simulink model "dynamic_calc"  (R2022b)
settings: Solver=VariableStepAuto  StartTime=0.0  StopTime=10.0  RelTol=1e-3
undefined symbols (not defined in the file): alfa_1, gravity_acceleration, i, Malpha, Malphadot, MdeltaE, Mq, Mtalpha, Mtu, Mu, o, Vp1, Xalpha, XdeltaE, Xtu, Xu, Zalpha, Zalphadot, ZdeltaE, Zq, Zu
libraries: simulink_extras x3
settings Model: Creator=48519  LastModifiedBy=48519

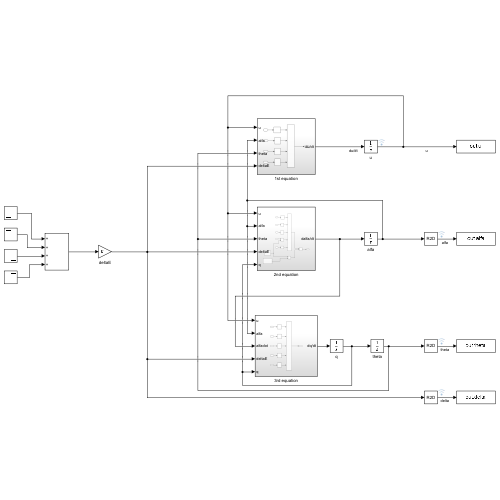
[thumbnail: Simulink's stored preview of the top-level diagram]
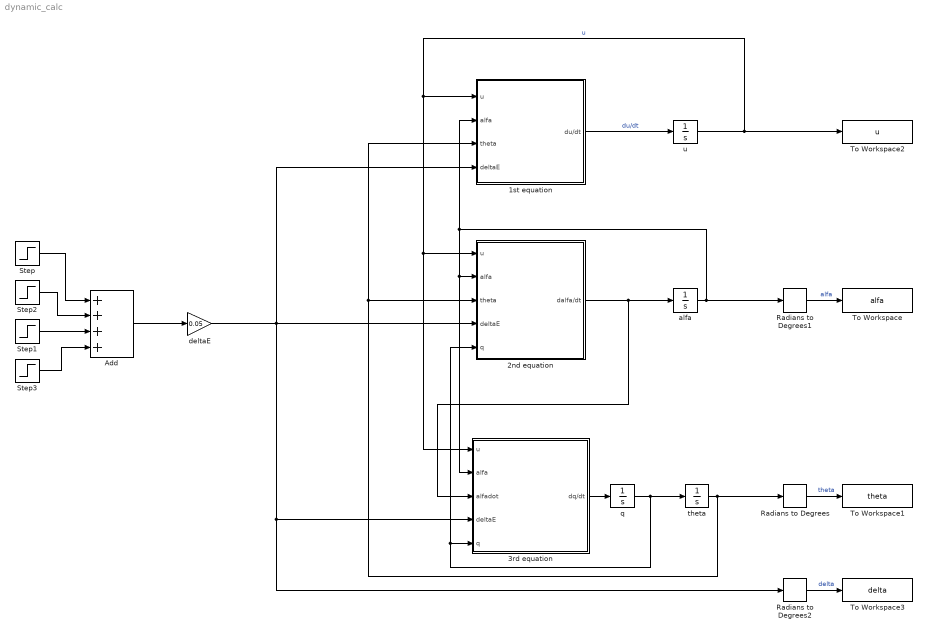
== system dynamic_calc ==
  1st equation : Subsystem
  2nd equation : Subsystem
  3rd equation : Subsystem
  Add : Sum  Inputs=++++
  Radians to Degrees : simulink_extras/Transformations/Radians to Degrees
  Radians to Degrees1 : simulink_extras/Transformations/Radians to Degrees
  Radians to Degrees2 : simulink_extras/Transformations/Radians to Degrees
  Step : Step  Time=2  SampleTime=0
  Step1 : Step  Time=62  After=-1  SampleTime=0
  Step2 : Step  Time=7  After=-1  SampleTime=0
  Step3 : Step  Time=67  SampleTime=0
  To Workspace : ToWorkspace  VariableName=alfa  SaveFormat=Timeseries  SampleTime=-1
  To Workspace1 : ToWorkspace  VariableName=theta  SaveFormat=Timeseries  SampleTime=-1
  To Workspace2 : ToWorkspace  VariableName=u  SaveFormat=Timeseries  SampleTime=-1
  To Workspace3 : ToWorkspace  VariableName=delta  SaveFormat=Timeseries  SampleTime=-1
  alfa : Integrator
  deltaE : Gain  Gain=0.05
  q : Integrator
  theta : Integrator
  u : Integrator
  wires:
  Radians to Degrees/1 -> To Workspace1/1  "theta"
  Radians to Degrees2/1 -> To Workspace3/1  "delta"
  theta/1 -> Radians to Degrees/1, 1st equation/3(theta), 2nd equation/3(theta)
  1st equation/1(du/dt) -> u/1  "du/dt"
  alfa/1 -> 3rd equation/2(alfa), 2nd equation/2(alfa), 1st equation/2(alfa), Radians to Degrees1/1
  Step1/1 -> Add/3
  deltaE/1 -> Radians to Degrees2/1, 3rd equation/4(deltaE), 1st equation/4(deltaE), 2nd equation/4(deltaE)
  3rd equation/1(dq/dt) -> q/1
  Step2/1 -> Add/2
  Step/1 -> Add/1
  u/1 -> 2nd equation/1(u), 3rd equation/1(u), 1st equation/1(u), To Workspace2/1  "u"
  Radians to Degrees1/1 -> To Workspace/1  "alfa"
  Step3/1 -> Add/4
  Add/1 -> deltaE/1
  q/1 -> theta/1, 3rd equation/5(q), 2nd equation/5(q)
  2nd equation/1(dalfa/dt) -> 3rd equation/3(alfadot), alfa/1

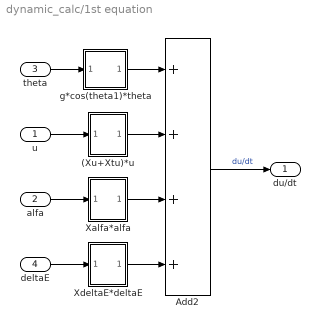
== system dynamic_calc/1st equation ==
  u : Inport
  alfa : Inport  Port=2
  theta : Inport  Port=3
  deltaE : Inport  Port=4
  (Xu+Xtu)*u : Subsystem
  Add2 : Sum  Inputs=++++
  Xalfa*alfa : Subsystem
  XdeltaE*deltaE : Subsystem
  g*cos(theta1)*theta : Subsystem
  du/dt : Outport
  wires:
  Add2/1 -> du/dt/1  "du/dt"
  theta/1 -> g*cos(theta1)*theta/1(theta)
  g*cos(theta1)*theta/1(Out1) -> Add2/1
  u/1 -> (Xu+Xtu)*u/1(In2)
  (Xu+Xtu)*u/1(Out1) -> Add2/2
  alfa/1 -> Xalfa*alfa/1(In1)
  Xalfa*alfa/1(Out1) -> Add2/3
  deltaE/1 -> XdeltaE*deltaE/1(In1)
  XdeltaE*deltaE/1(Out1) -> Add2/4

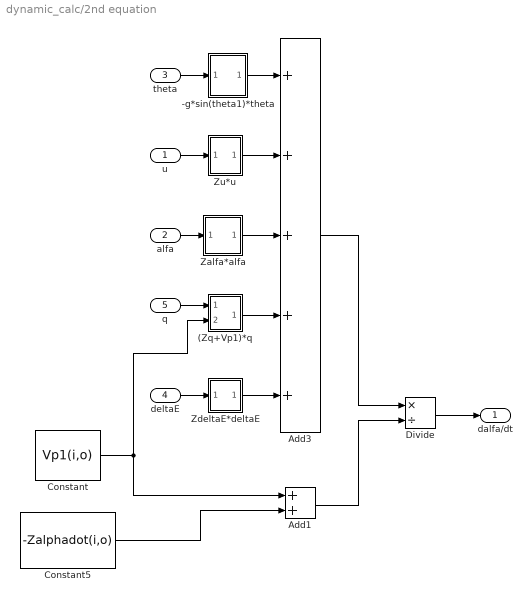
== system dynamic_calc/2nd equation ==
  u : Inport
  alfa : Inport  Port=2
  theta : Inport  Port=3
  deltaE : Inport  Port=4
  q : Inport  Port=5
  (Zq+Vp1)*q : Subsystem
  -g*sin(theta1)*theta : Subsystem
  Add1 : Sum
  Add3 : Sum  Inputs=+++++
  Constant : Constant  Value=Vp1(i,o)
  Constant5 : Constant  Value=-Zalphadot(i,o)
  Divide : Product  Inputs=*/
  Zalfa*alfa : Subsystem
  ZdeltaE*deltaE : Subsystem
  Zu*u : Subsystem
  dalfa/dt : Outport
  wires:
  Constant5/1 -> Add1/2
  Constant/1 -> Add1/1, (Zq+Vp1)*q/2(In2)
  Add3/1 -> Divide/1
  Add1/1 -> Divide/2
  Divide/1 -> dalfa/dt/1
  theta/1 -> -g*sin(theta1)*theta/1(In3)
  -g*sin(theta1)*theta/1(Out1) -> Add3/1
  u/1 -> Zu*u/1(In2)
  Zu*u/1(Out1) -> Add3/2
  alfa/1 -> Zalfa*alfa/1(In1)
  Zalfa*alfa/1(Out1) -> Add3/3
  q/1 -> (Zq+Vp1)*q/1(In5)
  (Zq+Vp1)*q/1(Out1) -> Add3/4
  deltaE/1 -> ZdeltaE*deltaE/1(In4)
  ZdeltaE*deltaE/1(Out1) -> Add3/5

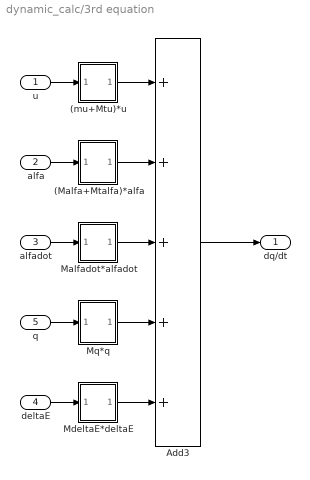
== system dynamic_calc/3rd equation ==
  u : Inport
  alfa : Inport  Port=2
  alfadot : Inport  Port=3
  deltaE : Inport  Port=4
  q : Inport  Port=5
  (Malfa+Mtalfa)*alfa : Subsystem
  (mu+Mtu)*u : Subsystem
  Add3 : Sum  Inputs=+++++
  Malfadot*alfadot : Subsystem
  MdeltaE*deltaE : Subsystem
  Mq*q : Subsystem
  dq/dt : Outport
  wires:
  Add3/1 -> dq/dt/1
  u/1 -> (mu+Mtu)*u/1(In1)
  (mu+Mtu)*u/1(Out1) -> Add3/1
  alfa/1 -> (Malfa+Mtalfa)*alfa/1(In3)
  (Malfa+Mtalfa)*alfa/1(Out1) -> Add3/2
  alfadot/1 -> Malfadot*alfadot/1(In2)
  Malfadot*alfadot/1(Out1) -> Add3/3
  q/1 -> Mq*q/1(In5)
  Mq*q/1(Out1) -> Add3/4
  deltaE/1 -> MdeltaE*deltaE/1(In4)
  MdeltaE*deltaE/1(Out1) -> Add3/5

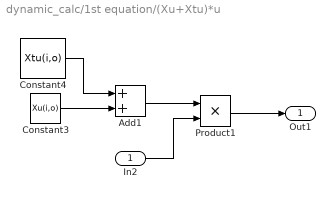
== system dynamic_calc/1st equation/(Xu+Xtu)*u ==
  In2 : Inport
  Add1 : Sum
  Constant3 : Constant  Value=Xu(i,o)
  Constant4 : Constant  Value=Xtu(i,o)
  Product1 : Product
  Out1 : Outport
  wires:
  Constant3/1 -> Add1/2
  Product1/1 -> Out1/1
  Constant4/1 -> Add1/1
  In2/1 -> Product1/2
  Add1/1 -> Product1/1

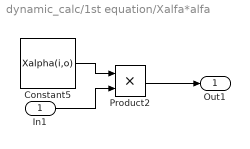
== system dynamic_calc/1st equation/Xalfa*alfa ==
  In1 : Inport
  Constant5 : Constant  Value=Xalpha(i,o)
  Product2 : Product
  Out1 : Outport
  wires:
  Constant5/1 -> Product2/1
  Product2/1 -> Out1/1
  In1/1 -> Product2/2

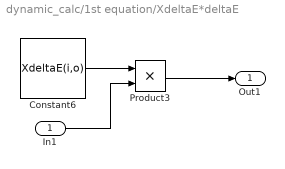
== system dynamic_calc/1st equation/XdeltaE*deltaE ==
  In1 : Inport
  Constant6 : Constant  Value=XdeltaE(i,o)
  Product3 : Product
  Out1 : Outport
  wires:
  Constant6/1 -> Product3/1
  Product3/1 -> Out1/1
  In1/1 -> Product3/2

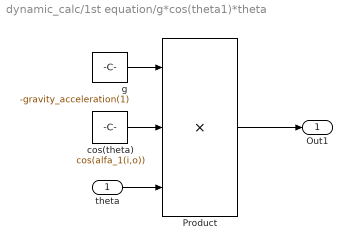
== system dynamic_calc/1st equation/g*cos(theta1)*theta ==
  theta : Inport
  Product : Product  Inputs=3
  cos(theta) : Constant  Value=cos(alfa_1(i,o))
  g : Constant  Value=-gravity_acceleration(1)
  Out1 : Outport
  wires:
  Product/1 -> Out1/1
  g/1 -> Product/1
  theta/1 -> Product/3
  cos(theta)/1 -> Product/2

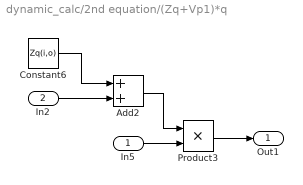
== system dynamic_calc/2nd equation/(Zq+Vp1)*q ==
  In5 : Inport
  In2 : Inport  Port=2
  Add2 : Sum
  Constant6 : Constant  Value=Zq(i,o)
  Product3 : Product
  Out1 : Outport
  wires:
  In2/1 -> Add2/2
  Add2/1 -> Product3/1
  Constant6/1 -> Add2/1
  In5/1 -> Product3/2
  Product3/1 -> Out1/1

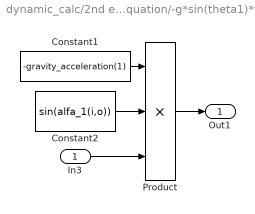
== system dynamic_calc/2nd equation/-g*sin(theta1)*theta ==
  In3 : Inport
  Constant1 : Constant  Value=-gravity_acceleration(1)
  Constant2 : Constant  Value=sin(alfa_1(i,o))
  Product : Product  Inputs=3
  Out1 : Outport
  wires:
  Constant2/1 -> Product/2
  Constant1/1 -> Product/1
  In3/1 -> Product/3
  Product/1 -> Out1/1

== system dynamic_calc/2nd equation/Zalfa*alfa ==
  In1 : Inport
  Constant4 : Constant  Value=Zalpha(i,o)
  Product2 : Product
  Out1 : Outport
  wires:
  Constant4/1 -> Product2/1
  In1/1 -> Product2/2
  Product2/1 -> Out1/1

== system dynamic_calc/2nd equation/ZdeltaE*deltaE ==
  In4 : Inport
  Constant7 : Constant  Value=ZdeltaE(i,o)
  Product4 : Product
  Out1 : Outport
  wires:
  Constant7/1 -> Product4/1
  In4/1 -> Product4/2
  Product4/1 -> Out1/1

== system dynamic_calc/2nd equation/Zu*u ==
  In2 : Inport
  Constant3 : Constant  Value=Zu(i,o)
  Product1 : Product
  Out1 : Outport
  wires:
  Constant3/1 -> Product1/1
  In2/1 -> Product1/2
  Product1/1 -> Out1/1

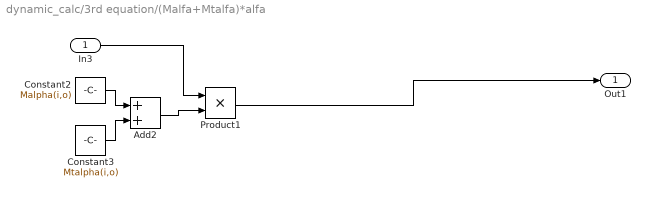
== system dynamic_calc/3rd equation/(Malfa+Mtalfa)*alfa ==
  In3 : Inport
  Add2 : Sum
  Constant2 : Constant  Value=Malpha(i,o)
  Constant3 : Constant  Value=Mtalpha(i,o)
  Product1 : Product
  Out1 : Outport
  wires:
  Constant2/1 -> Add2/1
  In3/1 -> Product1/1
  Constant3/1 -> Add2/2
  Product1/1 -> Out1/1
  Add2/1 -> Product1/2

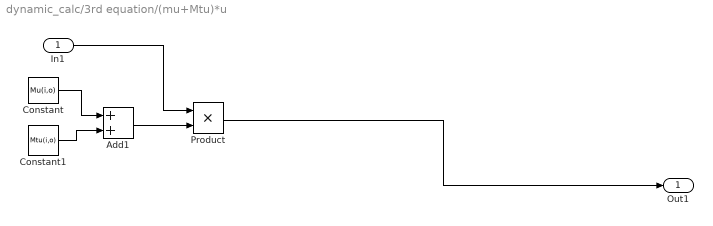
== system dynamic_calc/3rd equation/(mu+Mtu)*u ==
  In1 : Inport
  Add1 : Sum
  Constant : Constant  Value=Mu(i,o)
  Constant1 : Constant  Value=Mtu(i,o)
  Product : Product
  Out1 : Outport
  wires:
  Constant1/1 -> Add1/2
  Constant/1 -> Add1/1
  Add1/1 -> Product/2
  In1/1 -> Product/1
  Product/1 -> Out1/1

== system dynamic_calc/3rd equation/Malfadot*alfadot ==
  In2 : Inport
  Constant4 : Constant  Value=Malphadot(i,o)
  Product2 : Product
  Out1 : Outport
  wires:
  Constant4/1 -> Product2/2
  In2/1 -> Product2/1
  Product2/1 -> Out1/1

== system dynamic_calc/3rd equation/MdeltaE*deltaE ==
  In4 : Inport
  Constant6 : Constant  Value=MdeltaE(i,o)
  Product4 : Product
  Out1 : Outport
  wires:
  Constant6/1 -> Product4/2
  In4/1 -> Product4/1
  Product4/1 -> Out1/1

== system dynamic_calc/3rd equation/Mq*q ==
  In5 : Inport
  Constant5 : Constant  Value=Mq(i,o)
  Product3 : Product
  Out1 : Outport
  wires:
  In5/1 -> Product3/1
  Product3/1 -> Out1/1
  Constant5/1 -> Product3/2
